simulink model "springMassdamper"  (R2024b)
settings: Solver=VariableStepAuto  StartTime=0.0  StopTime=100  RelTol=1e-3
undefined symbols (not defined in the file): b, k, M

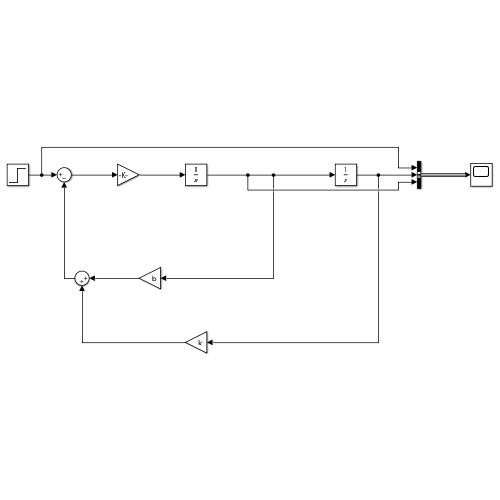
[thumbnail: Simulink's stored preview of the top-level diagram]
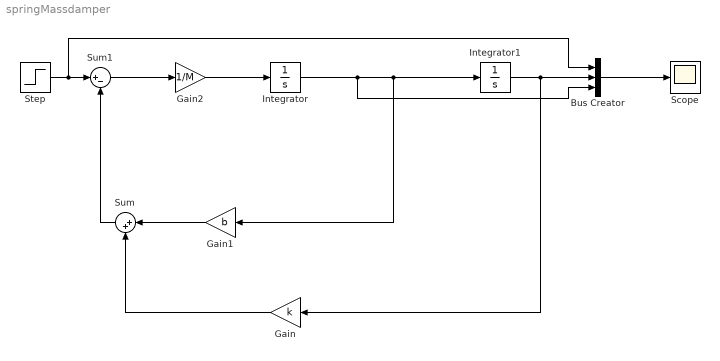
== system springMassdamper ==
  Bus Creator : BusCreator  Inputs=3
  Gain : Gain  Gain=k
  Gain1 : Gain  Gain=b
  Gain2 : Gain  Gain=1/M
  Integrator : Integrator
  Integrator1 : Integrator
  Scope : Scope
  Step : Step  SampleTime=0
  Sum : Sum  Inputs=|++
  Sum1 : Sum  Inputs=|+-
  wires:
  Integrator/1 -> Bus Creator/3, Gain1/1, Integrator1/1
  Integrator1/1 -> Bus Creator/2, Gain/1
  Gain1/1 -> Sum/1
  Gain/1 -> Sum/2
  Sum/1 -> Sum1/2
  Step/1 -> Bus Creator/1, Sum1/1
  Sum1/1 -> Gain2/1
  Gain2/1 -> Integrator/1
  Bus Creator/1 -> Scope/1
